simulink model "otobus_model"  (Simulink 7.6)
settings: Solver=ode45  StartTime=0.0  StopTime=64  FixedStep=0.00006  RelTol=1e-3
values from neighbouring files (symbols this model uses):
  cot1 = 6500    [bus.m]    (also in bus_sis.m)
  cot2 = 6500    [bus.m]    (also in bus_sis.m)
  cot3 = 6500    [bus.m]    (also in bus_sis.m)
  cot4 = 6500    [bus.m]    (also in bus_sis.m)
  cot5 = 6500    [bus.m]    (also in bus_sis.m)
  cot6 = 6500    [bus.m]    (also in bus_sis.m)
  dyot = 0.007    [bus.m]    (also in bus_sis.m)
  kot1 = 72000    [bus.m]    (also in bus_sis.m)
  kot10 = 921607    [bus.m]    (also in bus_sis.m)
  kot11 = 190000    [bus.m]    (also in bus_sis.m)
  kot12 = 921607    [bus.m]    (also in bus_sis.m)
  kot2 = 921607    [bus.m]    (also in bus_sis.m)
  kot3 = 190000    [bus.m]    (also in bus_sis.m)
  kot4 = 921607    [bus.m]    (also in bus_sis.m)
  kot5 = 190000    [bus.m]    (also in bus_sis.m)
  kot6 = 921607    [bus.m]    (also in bus_sis.m)
  kot7 = 72000    [bus.m]    (also in bus_sis.m)
  kot8 = 921607    [bus.m]    (also in bus_sis.m)
  kot9 = 190000    [bus.m]    (also in bus_sis.m)
  Lot1 = 3.812    [bus.m]    (also in bus_sis.m)
  Lot2 = 5.042    [bus.m]    (also in bus_sis.m)
  Lot3 = 0.84    [bus.m]    (also in bus_sis.m)
  Lot4 = 1.2    [bus.m]    (also in bus_sis.m)
  Lot5 = 1.2    [bus.m]    (also in bus_sis.m)
  mot2 = 1250    [bus.m]    (also in bus_sis.m)
  mot3 = 700    [bus.m]    (also in bus_sis.m)
  mot4 = 1250    [bus.m]    (also in bus_sis.m)
  mot5 = 1250    [bus.m]    (also in bus_sis.m)
  mot6 = 700    [bus.m]    (also in bus_sis.m)
  mot7 = 1250    [bus.m]    (also in bus_sis.m)
  Vot = 31.25    [bus.m]    (also in bus_sis.m = 16.6666666667)
  wot = Vot/dyot    (= 4464.28571429)    [bus.m]    (also in bus_sis.m = 2380.95238095)
settings Model: Creator=aster  LastModifiedBy=user
settings SolverCC: NumberNewtonIterations=100  ZeroCrossAlgorithm=Adaptive
settings OptimizationCC: InitFltsAndDblsToZero=on
settings DebuggingCC: StrictBusMsg=Warning

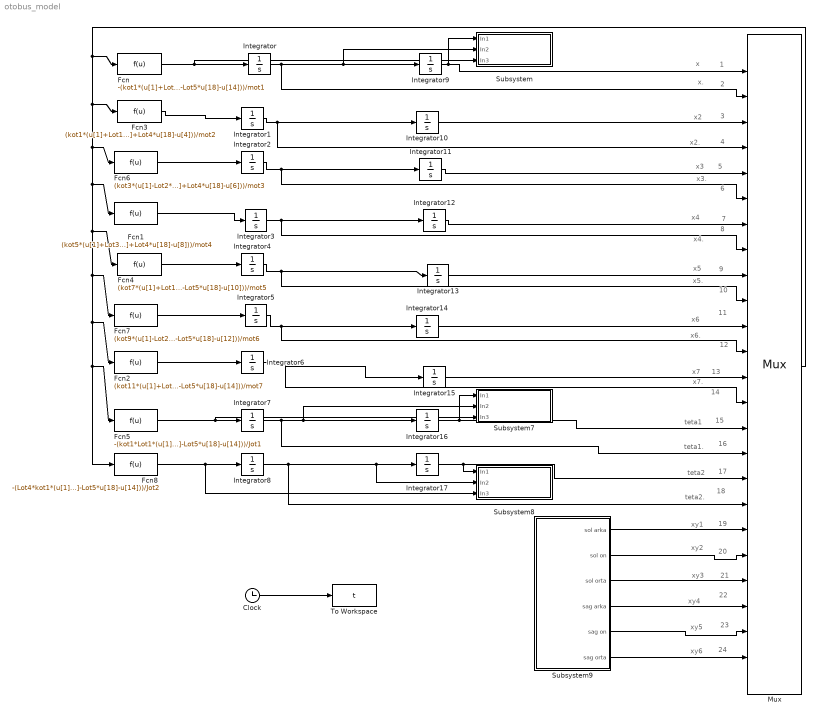
== system otobus_model ==
  note: x
  note: x.
  note: x2
  note: x2.
  note: x3
  note: x3.
  note: x4
  note: x4.
  note: x5
  note: x5.
  note: x6
  note: x6.
  note: x7
  note: x7.
  note: teta1
  note: teta1.
  note: teta2
  note: teta2.
  note: xy1
  note: xy2
  note: xy3
  note: xy4
  note: xy5
  note: xy6
  note: 1
  note: 2
  note: 3
  note: 4
  note: 5
  note: 6
  note: 7
  note: 8
  note: 9
  note: 10
  note: 11
  note: 12
  note: 13
  note: 14
  note: 15
  note: 16
  note: 17
  note: 18
  note: 19
  note: 20
  note: 21
  note: 22
  note: 23
  note: 24
  Clock : Clock
      settings: Decimation=10
  Fcn : Fcn  Expr=-(kot1*(u[1]+Lot1*u[15]+Lot4*u[17]-u[3])+kot3*(u[1]-Lot2*u[15]+Lot4*u[17]-u[5])+kot5*(u[1]+Lot3*u[15]+Lot4*u[17]-u[7])+kot7*(u[1]+Lot1*u[15]-Lot5*u[17]-u[9])+kot9*(u[1]-Lot2*u[15]-Lot5*u[17]-u[11])+kot11*(u[1]+Lot3*u[15]-Lot5*u[17]-u[13])+cot1*(u[2]+Lot1*u[16]+Lot4*u[18]-u[4])+cot2*(u[2]-Lot2*u[16]+Lot4*u[18]-u[6])+cot3*(u[2]+Lot3*u[16]+Lot4*u[18]-u[8])+cot4*(u[2]+Lot1*u[16]-Lot5*u[18]-u[10])+cot5*(u[2]-Lot2*u[16]-Lot5*u[18]-u[12])+cot6*(u[2]+Lot3*u[16]-Lot5*u[18]-u[14]))/mot1
  Fcn1 : Fcn  Expr=(kot5*(u[1]+Lot3*u[15]+Lot4*u[17]-u[7])-kot6*(u[7]-u[21])+cot3*(u[2]-Lot3*u[16]+Lot4*u[18]-u[8]))/mot4
  Fcn2 : Fcn  Expr=(kot11*(u[1]+Lot3*u[15]-Lot5*u[17]-u[13])-kot12*(u[13]-u[24])+cot6*(u[2]+Lot3*u[16]-Lot5*u[18]-u[14]))/mot7
  Fcn3 : Fcn  Expr=(kot1*(u[1]+Lot1*u[15]+Lot4*u[17]-u[3])-kot2*(u[3]-u[19])+cot1*(u[2]+Lot1*u[16]+Lot4*u[18]-u[4]))/mot2
  Fcn4 : Fcn  Expr=(kot7*(u[1]+Lot1*u[15]-Lot5*u[17]-u[9])-kot8*(u[9]-u[22])+cot4*(u[2]+Lot1*u[16]-Lot5*u[18]-u[10]))/mot5
  Fcn5 : Fcn  Expr=-(kot1*Lot1*(u[1]+Lot1*u[15]+Lot4*u[17]-u[3])-kot3*Lot2*(u[1]-Lot2*u[15]+Lot4*u[17]-u[5])+kot5*Lot3*(u[1]+Lot3*u[15]+Lot4*u[17]-u[7])+kot7*Lot1*(u[1]+Lot1*u[15]-Lot5*u[17]-u[9])-kot9*Lot2*(u[1]-Lot2*u[15]-Lot5*u[17]-u[11])+kot11*Lot3*(u[1]+Lot3*u[15]-Lot5*u[17]-u[13])+cot1*Lot1*(u[2]+Lot1*u[16]+Lot4*u[18]-u[4])-cot2*Lot2*(u[2]-Lot2*u[16]+Lot4*u[18]-u[6])+cot3*Lot3*(u[2]+Lot3*u[16]+Lot4*u[18]-u[8])+cot4*Lot1*(u[2]+Lot1*u[16]-Lot5*u[18]-u[10])-cot5*Lot2*(u[2]-Lot2*u[16]-Lot5*u[18]-u[12])+cot6*Lot3*(u[2]+Lot3*u[16]-Lot5*u[18]-u[14]))/Jot1
  Fcn6 : Fcn  Expr=(kot3*(u[1]-Lot2*u[15]+Lot4*u[17]-u[5])-kot4*(u[5]-u[20])+cot2*(u[2]-Lot2*u[16]+Lot4*u[18]-u[6]))/mot3
  Fcn7 : Fcn  Expr=(kot9*(u[1]-Lot2*u[15]-Lot5*u[17]-u[11])-kot10*(u[11]-u[23])+cot5*(u[2]-Lot2*u[16]-Lot5*u[18]-u[12]))/mot6
  Fcn8 : Fcn  Expr=-(Lot4*kot1*(u[1]+Lot1*u[15]+Lot4*u[17]-u[3])+Lot4*kot3*(u[1]-Lot2*u[15]+Lot4*u[17]-u[5])+Lot4*kot5*(u[1]+Lot3*u[15]+Lot4*u[17]-u[7])-Lot5*kot7*(u[1]+Lot1*u[15]-Lot5*u[17]-u[9])-Lot5*kot9*(u[1]-Lot2*u[15]-Lot5*u[17]-u[11])-Lot5*kot11*(u[1]+Lot3*u[15]-Lot5*u[17]-u[13])+Lot4*cot1*(u[2]+Lot1*u[16]+Lot4*u[18]-u[4])+Lot4*cot2*(u[2]-Lot2*u[16]+Lot4*u[18]-u[6])+Lot4*cot3*(u[2]+Lot3*u[16]+Lot4*u[18]-u[8])-Lot5*cot4*(u[2]+Lot1*u[16]-Lot5*u[18]-u[10])-Lot5*cot5*(u[2]-Lot2*u[16]-Lot5*u[18]-u[12])-Lot5*cot6*(u[2]+Lot3*u[16]-Lot5*u[18]-u[14]))/Jot2
  Integrator{,1..17} (18 alike) : Integrator
  Mux : Mux  Inputs=24
  Subsystem : Subsystem
  Subsystem7 : Subsystem
  Subsystem8 : Subsystem
  Subsystem9 : Subsystem
  To Workspace : ToWorkspace  VariableName=t  SampleTime=-1  SaveFormat=Array
  wires:
  Fcn/1 -> Integrator/1, Subsystem/3(In3)
  Fcn3/1 -> Integrator1/1
  Fcn6/1 -> Integrator2/1
  Fcn1/1 -> Integrator3/1
  Fcn4/1 -> Integrator4/1
  Fcn7/1 -> Integrator5/1
  Fcn2/1 -> Integrator6/1
  Fcn5/1 -> Integrator7/1, Subsystem7/3(In3)
  Fcn8/1 -> Integrator8/1, Subsystem8/3(In3)
  Integrator/1 -> Mux/2, Integrator9/1, Subsystem/2(In2)
  Integrator1/1 -> Mux/4, Integrator10/1
  Integrator2/1 -> Mux/6, Integrator11/1
  Integrator3/1 -> Mux/8, Integrator12/1
  Integrator4/1 -> Mux/10, Integrator13/1
  Integrator5/1 -> Mux/12, Integrator14/1
  Integrator6/1 -> Mux/14, Integrator15/1
  Integrator7/1 -> Mux/16, Integrator16/1, Subsystem7/2(In2)
  Integrator8/1 -> Mux/18, Integrator17/1, Subsystem8/2(In2)
  Mux/1 -> Fcn8/1, Fcn5/1, Fcn2/1, Fcn7/1, Fcn4/1, Fcn1/1, Fcn6/1, Fcn3/1, Fcn/1
  Integrator9/1 -> Subsystem/1(In1), Mux/1
  Integrator10/1 -> Mux/3
  Integrator11/1 -> Mux/5
  Integrator12/1 -> Mux/7
  Integrator13/1 -> Mux/9
  Integrator14/1 -> Mux/11
  Integrator15/1 -> Mux/13
  Integrator16/1 -> Mux/15, Subsystem7/1(In1)
  Integrator17/1 -> Mux/17, Subsystem8/1(In1)
  Clock/1 -> To Workspace/1
  Subsystem9/1(sol arka) -> Mux/19
  Subsystem9/2(sol on) -> Mux/20
  Subsystem9/3(sol orta) -> Mux/21
  Subsystem9/4(sag arka) -> Mux/22
  Subsystem9/5(sag on) -> Mux/23
  Subsystem9/6(sag orta) -> Mux/24

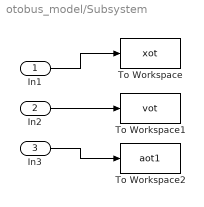
== system otobus_model/Subsystem ==
  In1 : Inport
  In2 : Inport  Port=2
  In3 : Inport  Port=3
  To Workspace : ToWorkspace  VariableName=xot  SampleTime=-1  SaveFormat=Array
  To Workspace1 : ToWorkspace  VariableName=vot  SampleTime=-1  SaveFormat=Array
  To Workspace2 : ToWorkspace  VariableName=aot1  SampleTime=-1  SaveFormat=Array
  wires:
  In1/1 -> To Workspace/1
  In2/1 -> To Workspace1/1
  In3/1 -> To Workspace2/1

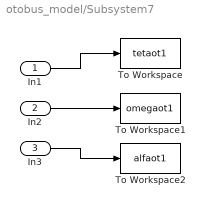
== system otobus_model/Subsystem7 ==
  In1 : Inport
  In2 : Inport  Port=2
  In3 : Inport  Port=3
  To Workspace : ToWorkspace  VariableName=tetaot1  SampleTime=-1  SaveFormat=Array
  To Workspace1 : ToWorkspace  VariableName=omegaot1  SampleTime=-1  SaveFormat=Array
  To Workspace2 : ToWorkspace  VariableName=alfaot1  SampleTime=-1  SaveFormat=Array
  wires:
  In3/1 -> To Workspace2/1
  In2/1 -> To Workspace1/1
  In1/1 -> To Workspace/1

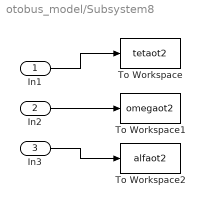
== system otobus_model/Subsystem8 ==
  In1 : Inport
  In2 : Inport  Port=2
  In3 : Inport  Port=3
  To Workspace : ToWorkspace  VariableName=tetaot2  SampleTime=-1  SaveFormat=Array
  To Workspace1 : ToWorkspace  VariableName=omegaot2  SampleTime=-1  SaveFormat=Array
  To Workspace2 : ToWorkspace  VariableName=alfaot2  SampleTime=-1  SaveFormat=Array
  wires:
  In1/1 -> To Workspace/1
  In2/1 -> To Workspace1/1
  In3/1 -> To Workspace2/1

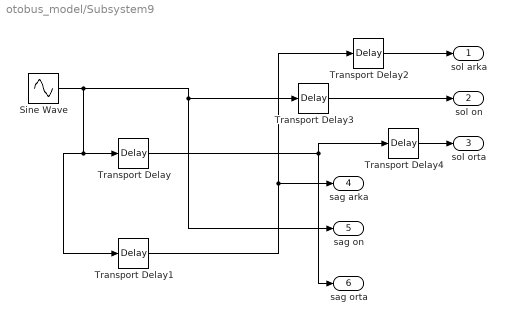
== system otobus_model/Subsystem9 ==
  Sine Wave : Sin  Amplitude=dyot  Frequency=wot*2*pi  SampleTime=0
  Transport Delay : TransportDelay  DelayTime=(Lot2+Lot3)/Vot
  Transport Delay1 : TransportDelay  DelayTime=(Lot1+Lot2)/Vot
  Transport Delay2 : TransportDelay  DelayTime=0.001
  Transport Delay3 : TransportDelay  DelayTime=0.001
  Transport Delay4 : TransportDelay  DelayTime=0.001
  sol arka : Outport
  sol on : Outport  Port=2
  sol orta : Outport  Port=3
  sag arka : Outport  Port=4
  sag on : Outport  Port=5
  sag orta : Outport  Port=6
  wires:
  Sine Wave/1 -> sag on/1, Transport Delay3/1, Transport Delay/1, Transport Delay1/1
  Transport Delay/1 -> sag orta/1, Transport Delay4/1
  Transport Delay1/1 -> sag arka/1, Transport Delay2/1
  Transport Delay2/1 -> sol arka/1
  Transport Delay3/1 -> sol on/1
  Transport Delay4/1 -> sol orta/1
